simulink model "sensorless"  (R2018b)
settings: Solver=ode45  StartTime=0.0  StopTime=0.5  RelTol=1e-3  EnableMultiTasking=on
InitFcn:
  | tpwm=0.0001;
  | K=0.0604;
  | L1=0.00248;
  | L2=-1.239e-7*40;
  | Td=0;
  | kr=50;
  | wc=5;
  | speedref=10;
  | L1=0.00248;
  | L2=-1.239e-7*200;
libraries: dspsigops x72, powerlib x31, powerlib_meascontrol x24, simulink x8, powerlib_extras x5
(part 2 of 2)

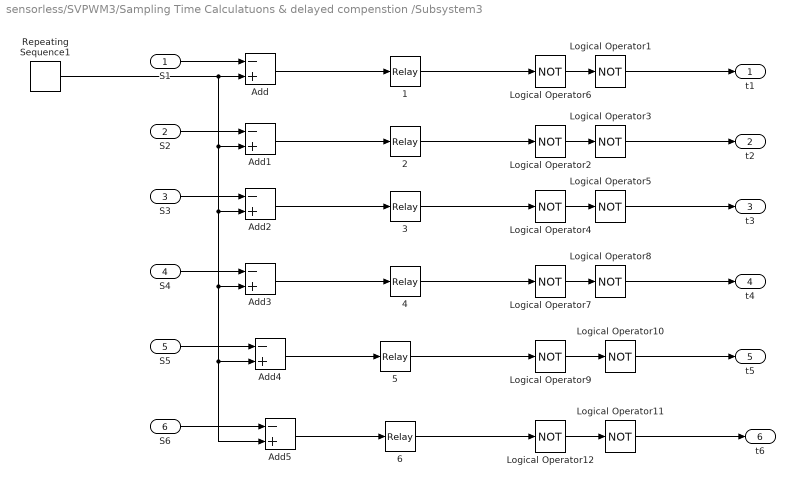
== system sensorless/SVPWM3/Sampling Time Calculatuons & delayed compenstion /Subsystem3 ==
  S1 : Inport
  S2 : Inport  Port=2
  S3 : Inport  Port=3
  S4 : Inport  Port=4
  S5 : Inport  Port=5
  S6 : Inport  Port=6
  {1..6} (6 alike) : Relay
  Add{,1..5} (6 alike) : Sum  Inputs=-+
  Logical Operator{1..12} (12 alike) : Logic  Operator=NOT  AllPortsSameDT=off  OutDataTypeStr=boolean
  Repeating Sequence1 : simulink/Sources/Repeating Sequence  rep_seq_t=[0 tpwm]  rep_seq_y=[0 tpwm]
  t1 : Outport
  t2 : Outport  Port=2
  t3 : Outport  Port=3
  t4 : Outport  Port=4
  t5 : Outport  Port=5
  t6 : Outport  Port=6
  wires:
  Add/1 -> 1/1
  1/1 -> Logical Operator6/1
  Logical Operator6/1 -> Logical Operator1/1
  Logical Operator2/1 -> Logical Operator3/1
  S1/1 -> Add/1
  S2/1 -> Add1/1
  S3/1 -> Add2/1
  Logical Operator4/1 -> Logical Operator5/1
  Add1/1 -> 2/1
  Add2/1 -> 3/1
  2/1 -> Logical Operator2/1
  3/1 -> Logical Operator4/1
  Logical Operator3/1 -> t2/1
  Logical Operator5/1 -> t3/1
  Logical Operator1/1 -> t1/1
  S4/1 -> Add3/1
  Add3/1 -> 4/1
  4/1 -> Logical Operator7/1
  Logical Operator7/1 -> Logical Operator8/1
  Logical Operator8/1 -> t4/1
  S5/1 -> Add4/1
  Add4/1 -> 5/1
  5/1 -> Logical Operator9/1
  Logical Operator9/1 -> Logical Operator10/1
  Logical Operator10/1 -> t5/1
  S6/1 -> Add5/1
  Add5/1 -> 6/1
  6/1 -> Logical Operator12/1
  Logical Operator12/1 -> Logical Operator11/1
  Logical Operator11/1 -> t6/1
  Repeating Sequence1/1 -> Add3/2, Add4/2, Add5/2, Add2/2, Add1/2, Add/2

== system sensorless/SVPWM3/Subsystem/Subsystem1 ==
  t1 : Inport
  t2 : Inport  Port=2
  tpwm : Inport  Port=3
  dt1 : Inport  Port=4
  phase currents : Inport  Port=5
  Add{,1..5} (6 alike) : Sum  Inputs=-+
  Divide{1..6} (6 alike) : Product  Inputs=*/
  PWM7 : Scope  NumInputPorts=2
  Sampled Current @ t2 : Subsystem
  Sampled Currents @ t1 : Subsystem
  Out1 : Outport
  Out2 : Outport  Port=2
  Out3 : Outport  Port=3
  Out4 : Outport  Port=4
  Out5 : Outport  Port=5
  Out6 : Outport  Port=6
  wires:
  Divide6/1 -> Out6/1
  Divide5/1 -> Out5/1
  Divide4/1 -> Out4/1
  Divide3/1 -> Out3/1
  Divide2/1 -> Out2/1
  Divide1/1 -> PWM7/1, Out1/1
  t2/1 -> Sampled Current @ t2/1(t1)
  t1/1 -> Sampled Currents @ t1/1(t1)
  phase currents/1 -> Sampled Currents @ t1/3(phase currents), Sampled Current @ t2/2(phase currents)
  tpwm/1 -> Sampled Currents @ t1/2(tpwm), Sampled Current @ t2/3(tpwm)
  dt1/1 -> Divide6/2, Divide5/2, Divide4/2, Divide3/2, Divide2/2, Divide1/2
  Add4/1 -> Divide5/1
  Add3/1 -> Divide4/1
  Sampled Current @ t2/6(Out6) -> Add5/2
  Sampled Current @ t2/2(Out2) -> Add1/2
  Add2/1 -> Divide3/1
  Sampled Currents @ t1/5(Out5) -> Add4/1
  Sampled Currents @ t1/4(Out4) -> Add3/1
  Sampled Current @ t2/5(Out5) -> Add4/2
  Add1/1 -> Divide2/1
  Sampled Current @ t2/4(Out4) -> Add3/2
  Sampled Currents @ t1/6(Out6) -> Add5/1
  Sampled Currents @ t1/1(Out1) -> Add/1
  Sampled Currents @ t1/3(Out3) -> Add2/1
  Add/1 -> Divide1/1, PWM7/2
  Sampled Current @ t2/1(Out1) -> Add/2
  Sampled Currents @ t1/2(Out2) -> Add1/1
  Add5/1 -> Divide6/1
  Sampled Current @ t2/3(Out3) -> Add2/2

== system sensorless/SVPWM3/Subsystem/Subsystem3 ==
  t1 : Inport
  t2 : Inport  Port=2
  tpwm : Inport  Port=3
  dt1 : Inport  Port=4
  phase currents : Inport  Port=5
  Add{,1..5} (6 alike) : Sum  Inputs=-+
  Divide{1..6} (6 alike) : Product  Inputs=*/
  PWM7 : Scope  NumInputPorts=2
  Sampled Current @ t2 : Subsystem
  Sampled Currents @ t1 : Subsystem
  Out1 : Outport
  Out2 : Outport  Port=2
  Out3 : Outport  Port=3
  Out4 : Outport  Port=4
  Out5 : Outport  Port=5
  Out6 : Outport  Port=6
  wires:
  Sampled Current @ t2/3(Out3) -> Add2/2
  Add5/1 -> Divide6/1
  Sampled Currents @ t1/2(Out2) -> Add1/1
  Sampled Current @ t2/1(Out1) -> Add/2
  Add/1 -> PWM7/2, Divide1/1
  Sampled Currents @ t1/3(Out3) -> Add2/1
  Sampled Currents @ t1/1(Out1) -> Add/1
  Sampled Currents @ t1/6(Out6) -> Add5/1
  Sampled Current @ t2/4(Out4) -> Add3/2
  Add1/1 -> Divide2/1
  Sampled Current @ t2/5(Out5) -> Add4/2
  Sampled Currents @ t1/4(Out4) -> Add3/1
  Sampled Currents @ t1/5(Out5) -> Add4/1
  Add2/1 -> Divide3/1
  Sampled Current @ t2/2(Out2) -> Add1/2
  Sampled Current @ t2/6(Out6) -> Add5/2
  Add3/1 -> Divide4/1
  Add4/1 -> Divide5/1
  dt1/1 -> Divide1/2, Divide2/2, Divide3/2, Divide4/2, Divide5/2, Divide6/2
  tpwm/1 -> Sampled Current @ t2/3(tpwm), Sampled Currents @ t1/2(tpwm)
  phase currents/1 -> Sampled Current @ t2/2(phase currents), Sampled Currents @ t1/3(phase currents)
  t1/1 -> Sampled Currents @ t1/1(t1)
  t2/1 -> Sampled Current @ t2/1(t1)
  Divide1/1 -> Out1/1, PWM7/1
  Divide2/1 -> Out2/1
  Divide3/1 -> Out3/1
  Divide4/1 -> Out4/1
  Divide5/1 -> Out5/1
  Divide6/1 -> Out6/1

== system sensorless/SVPWM3/Subsystem/Subsystem4 ==
  t1 : Inport
  t2 : Inport  Port=2
  tpwm : Inport  Port=3
  dt1 : Inport  Port=4
  phase currents : Inport  Port=5
  Add{,1..5} (6 alike) : Sum  Inputs=-+
  Divide{1..6} (6 alike) : Product  Inputs=*/
  PWM7 : Scope  NumInputPorts=2
  Sampled Current @ t2 : Subsystem
  Sampled Currents @ t1 : Subsystem
  Out1 : Outport
  Out2 : Outport  Port=2
  Out3 : Outport  Port=3
  Out4 : Outport  Port=4
  Out5 : Outport  Port=5
  Out6 : Outport  Port=6
  wires:
  Sampled Current @ t2/3(Out3) -> Add2/2
  Add5/1 -> Divide6/1
  Sampled Currents @ t1/2(Out2) -> Add1/1
  Sampled Current @ t2/1(Out1) -> Add/2
  Add/1 -> PWM7/2, Divide1/1
  Sampled Currents @ t1/3(Out3) -> Add2/1
  Sampled Currents @ t1/1(Out1) -> Add/1
  Sampled Currents @ t1/6(Out6) -> Add5/1
  Sampled Current @ t2/4(Out4) -> Add3/2
  Add1/1 -> Divide2/1
  Sampled Current @ t2/5(Out5) -> Add4/2
  Sampled Currents @ t1/4(Out4) -> Add3/1
  Sampled Currents @ t1/5(Out5) -> Add4/1
  Add2/1 -> Divide3/1
  Sampled Current @ t2/2(Out2) -> Add1/2
  Sampled Current @ t2/6(Out6) -> Add5/2
  Add3/1 -> Divide4/1
  Add4/1 -> Divide5/1
  dt1/1 -> Divide1/2, Divide2/2, Divide3/2, Divide4/2, Divide5/2, Divide6/2
  tpwm/1 -> Sampled Current @ t2/3(tpwm), Sampled Currents @ t1/2(tpwm)
  phase currents/1 -> Sampled Current @ t2/2(phase currents), Sampled Currents @ t1/3(phase currents)
  t1/1 -> Sampled Currents @ t1/1(t1)
  t2/1 -> Sampled Current @ t2/1(t1)
  Divide1/1 -> Out1/1, PWM7/1
  Divide2/1 -> Out2/1
  Divide3/1 -> Out3/1
  Divide4/1 -> Out4/1
  Divide5/1 -> Out5/1
  Divide6/1 -> Out6/1

== system sensorless/dq-sixphasePMSM/dynamics/Theta Generator (-pi, pi) ==
  pi : Inport
  In : Inport  Port=2
  Compare To Constant : simulink/Logic and Bit Operations/Compare To Constant  relop=>  const=pi/2  OutDataTypeStr=uint8  ZeroCross=off
  Constant3 : Constant  Value=0
  Sum2 : Sum  Inputs=+-
  Switch : Switch  Threshold=0.5
  Out : Outport
  wires:
  Compare To Constant/1 -> Switch/2
  Switch/1 -> Sum2/2
  Constant3/1 -> Switch/3
  pi/1 -> Switch/1
  In/1 -> Sum2/1, Compare To Constant/1
  Sum2/1 -> Out/1

== system sensorless/dq-sixphasePMSM/z-p/Subsystem ==
  Phase : Inport
  La0 : Constant  Value=-0.00139e-3
  La1 : Constant  Value=1.5201e-3
  La2 : Constant  Value=0.54985e-3
  Ldq_dmm1 : Scope  NumInputPorts=6
  Lg0 : Constant  Value=-0.0000798e-3
  Lg1 : Constant  Value=-0.000032e-3
  Lg2 : Constant  Value=-0.000052e-3
  "Manually Calculated Results " : MATLAB Function  TreatAsAtomicUnit=on
  Lz1 : Outport
  Lz2 : Outport  Port=2
  Lz1z2 : Outport  Port=3
  wires:
  "Manually Calculated Results "/3(Lz1) -> Lz1/1, Ldq_dmm1/3
  Lg2/1 -> "Manually Calculated Results "/6(Lg2)
  Lg1/1 -> "Manually Calculated Results "/5(Lg1)
  "Manually Calculated Results "/2(Lq) -> Ldq_dmm1/2
  Lg0/1 -> "Manually Calculated Results "/3(Lg0)
  "Manually Calculated Results "/4(Lz2) -> Lz2/1, Ldq_dmm1/4
  "Manually Calculated Results "/1(Ld) -> Ldq_dmm1/1
  "Manually Calculated Results "/5(Lz1z2) -> Lz1z2/1, Ldq_dmm1/5
  La0/1 -> "Manually Calculated Results "/1(La0)
  La1/1 -> "Manually Calculated Results "/2(La1)
  La2/1 -> "Manually Calculated Results "/4(La2)
  Phase/1 -> "Manually Calculated Results "/7(RP)

== system sensorless/dq-sixphasePMSM/z-p1/Subsystem ==
  Phase : Inport
  La0 : Constant  Value=-0.00139e-3
  La1 : Constant  Value=1.5201e-3
  La2 : Constant  Value=0.54985e-3
  Ldq_dmm1 : Scope  NumInputPorts=3
  Lg0 : Constant  Value=-0.0000798e-3
  Lg1 : Constant  Value=-0.000032e-3
  Lg2 : Constant  Value=-0.000052e-3
  "Manually Calculated Results " : MATLAB Function  TreatAsAtomicUnit=on
  Lalpha : Outport
  Lbeta : Outport  Port=2
  Lalpha_beta : Outport  Port=3
  wires:
  Lg2/1 -> "Manually Calculated Results "/6(Lg2)
  Lg1/1 -> "Manually Calculated Results "/5(Lg1)
  "Manually Calculated Results "/2(Lbeta) -> Ldq_dmm1/2, Lbeta/1
  Lg0/1 -> "Manually Calculated Results "/3(Lg0)
  "Manually Calculated Results "/1(Lalpha) -> Lalpha/1, Ldq_dmm1/1
  La0/1 -> "Manually Calculated Results "/1(La0)
  La1/1 -> "Manually Calculated Results "/2(La1)
  La2/1 -> "Manually Calculated Results "/4(La2)
  Phase/1 -> "Manually Calculated Results "/7(RP)
  "Manually Calculated Results "/3(Lalphabeta) -> Ldq_dmm1/3, Lalpha_beta/1

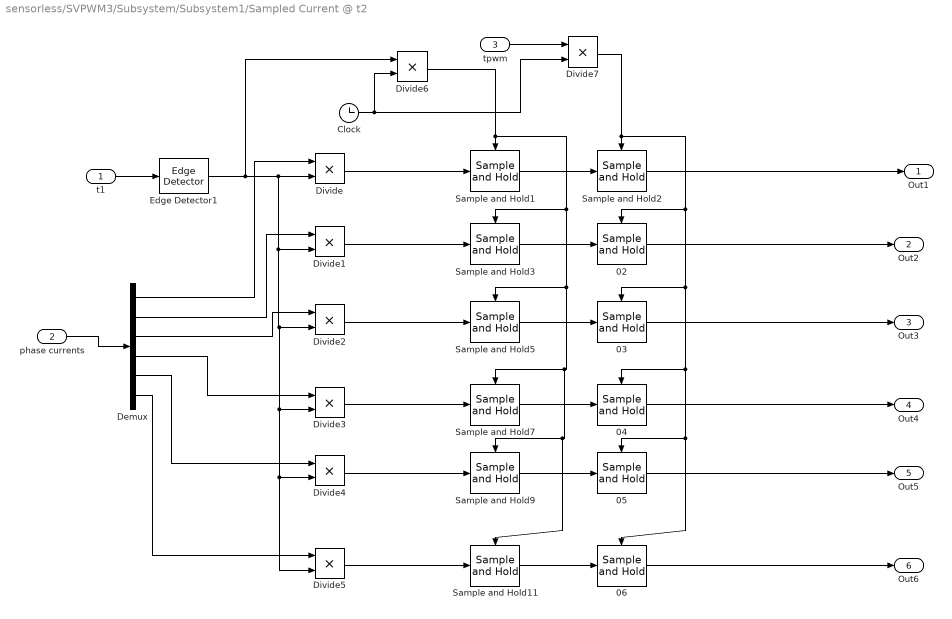
== system sensorless/SVPWM3/Subsystem/Subsystem1/Sampled Current @ t2 ==
  t1 : Inport
  phase currents : Inport  Port=2
  tpwm : Inport  Port=3
  02 : dspsigops/Sample and Hold  trig=Rising edge  initCond=0  latchinput=off
  03 : dspsigops/Sample and Hold  trig=Rising edge  initCond=0  latchinput=off
  04 : dspsigops/Sample and Hold  trig=Rising edge  initCond=0  latchinput=off
  "05 " : dspsigops/Sample and Hold  trig=Rising edge  initCond=0  latchinput=off
  06 : dspsigops/Sample and Hold  trig=Rising edge  initCond=0  latchinput=off
  Clock : Clock
  Demux : Demux  Outputs=6
  Divide{,1..7} (8 alike) : Product  Inputs=**
  Edge Detector1 : powerlib_meascontrol/Logic/Edge Detector  model=Rising  ic=0  Ts=0
      settings: SourceProductName=Simscape Power Systems  SourceProductBaseCode=PS
  Sample and Hold{1..3,5,7,9,11} (7 alike) : dspsigops/Sample and Hold  trig=Rising edge  initCond=0  latchinput=off
  Out1 : Outport
  Out2 : Outport  Port=2
  Out3 : Outport  Port=3
  Out4 : Outport  Port=4
  Out5 : Outport  Port=5
  Out6 : Outport  Port=6
  wires:
  Divide6/1 -> Sample and Hold11/Trigger, Sample and Hold9/Trigger, Sample and Hold7/Trigger, Sample and Hold5/Trigger, Sample and Hold3/Trigger, Sample and Hold1/Trigger
  06/1 -> Out6/1
  "05 "/1 -> Out5/1
  04/1 -> Out4/1
  03/1 -> Out3/1
  02/1 -> Out2/1
  Sample and Hold2/1 -> Out1/1
  Sample and Hold1/1 -> Sample and Hold2/1
  Edge Detector1/1 -> Divide6/1, Divide5/2, Divide4/2, Divide3/2, Divide2/2, Divide1/2, Divide/2
  Divide/1 -> Sample and Hold1/1
  t1/1 -> Edge Detector1/1
  Clock/1 -> Divide7/2, Divide6/2
  Divide7/1 -> 02/Trigger, 03/Trigger, 04/Trigger, "05 "/Trigger, 06/Trigger, Sample and Hold2/Trigger
  tpwm/1 -> Divide7/1
  Divide1/1 -> Sample and Hold3/1
  Sample and Hold3/1 -> 02/1
  Divide2/1 -> Sample and Hold5/1
  Sample and Hold5/1 -> 03/1
  Divide3/1 -> Sample and Hold7/1
  Sample and Hold7/1 -> 04/1
  Divide4/1 -> Sample and Hold9/1
  Sample and Hold9/1 -> "05 "/1
  Divide5/1 -> Sample and Hold11/1
  Sample and Hold11/1 -> 06/1
  phase currents/1 -> Demux/1
  Demux/1 -> Divide/1
  Demux/2 -> Divide1/1
  Demux/3 -> Divide2/1
  Demux/4 -> Divide3/1
  Demux/5 -> Divide4/1
  Demux/6 -> Divide5/1

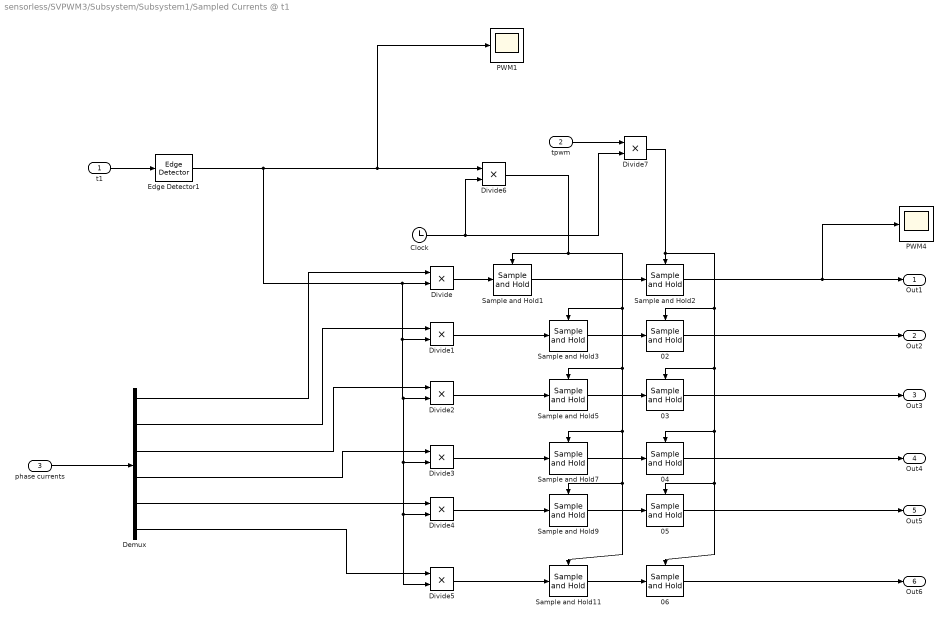
== system sensorless/SVPWM3/Subsystem/Subsystem1/Sampled Currents @ t1 ==
  t1 : Inport
  tpwm : Inport  Port=2
  phase currents : Inport  Port=3
  02 : dspsigops/Sample and Hold  trig=Rising edge  initCond=0  latchinput=off
  03 : dspsigops/Sample and Hold  trig=Rising edge  initCond=0  latchinput=off
  04 : dspsigops/Sample and Hold  trig=Rising edge  initCond=0  latchinput=off
  "05 " : dspsigops/Sample and Hold  trig=Rising edge  initCond=0  latchinput=off
  06 : dspsigops/Sample and Hold  trig=Rising edge  initCond=0  latchinput=off
  Clock : Clock
  Demux : Demux  Outputs=6
  Divide{,1..7} (8 alike) : Product  Inputs=**
  Edge Detector1 : powerlib_meascontrol/Logic/Edge Detector  model=Rising  ic=0  Ts=0
      settings: SourceProductName=Simscape Power Systems  SourceProductBaseCode=PS
  PWM1 : Scope
  PWM4 : Scope
  Sample and Hold{1..3,5,7,9,11} (7 alike) : dspsigops/Sample and Hold  trig=Rising edge  initCond=0  latchinput=off
  Out1 : Outport
  Out2 : Outport  Port=2
  Out3 : Outport  Port=3
  Out4 : Outport  Port=4
  Out5 : Outport  Port=5
  Out6 : Outport  Port=6
  wires:
  06/1 -> Out6/1
  "05 "/1 -> Out5/1
  04/1 -> Out4/1
  03/1 -> Out3/1
  02/1 -> Out2/1
  Sample and Hold2/1 -> PWM4/1, Out1/1
  Sample and Hold1/1 -> Sample and Hold2/1
  Divide/1 -> Sample and Hold1/1
  t1/1 -> Edge Detector1/1
  Clock/1 -> Divide6/2, Divide7/2
  Divide6/1 -> Sample and Hold11/Trigger, Sample and Hold9/Trigger, Sample and Hold7/Trigger, Sample and Hold5/Trigger, Sample and Hold3/Trigger, Sample and Hold1/Trigger
  tpwm/1 -> Divide7/1
  Divide1/1 -> Sample and Hold3/1
  Sample and Hold3/1 -> 02/1
  Divide2/1 -> Sample and Hold5/1
  Sample and Hold5/1 -> 03/1
  Divide3/1 -> Sample and Hold7/1
  Sample and Hold7/1 -> 04/1
  Divide4/1 -> Sample and Hold9/1
  Sample and Hold9/1 -> "05 "/1
  Divide5/1 -> Sample and Hold11/1
  Sample and Hold11/1 -> 06/1
  phase currents/1 -> Demux/1
  Demux/1 -> Divide/1
  Demux/2 -> Divide1/1
  Demux/3 -> Divide2/1
  Demux/4 -> Divide3/1
  Demux/5 -> Divide4/1
  Demux/6 -> Divide5/1
  Divide7/1 -> 02/Trigger, 03/Trigger, 04/Trigger, "05 "/Trigger, 06/Trigger, Sample and Hold2/Trigger
  Edge Detector1/1 -> Divide5/2, Divide4/2, Divide3/2, Divide2/2, Divide1/2, Divide/2, Divide6/1, PWM1/1

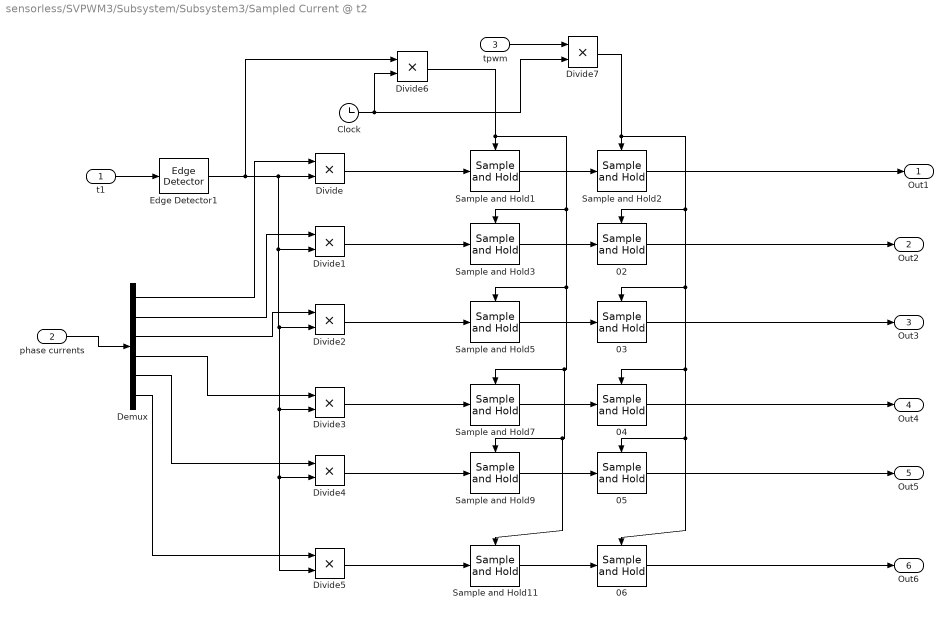
== system sensorless/SVPWM3/Subsystem/Subsystem3/Sampled Current @ t2 ==
  t1 : Inport
  phase currents : Inport  Port=2
  tpwm : Inport  Port=3
  02 : dspsigops/Sample and Hold  trig=Rising edge  initCond=0  latchinput=off
  03 : dspsigops/Sample and Hold  trig=Rising edge  initCond=0  latchinput=off
  04 : dspsigops/Sample and Hold  trig=Rising edge  initCond=0  latchinput=off
  "05 " : dspsigops/Sample and Hold  trig=Rising edge  initCond=0  latchinput=off
  06 : dspsigops/Sample and Hold  trig=Rising edge  initCond=0  latchinput=off
  Clock : Clock
  Demux : Demux  Outputs=6
  Divide{,1..7} (8 alike) : Product  Inputs=**
  Edge Detector1 : powerlib_meascontrol/Logic/Edge Detector  model=Rising  ic=0  Ts=0
      settings: SourceProductName=Simscape Power Systems  SourceProductBaseCode=PS
  Sample and Hold{1..3,5,7,9,11} (7 alike) : dspsigops/Sample and Hold  trig=Rising edge  initCond=0  latchinput=off
  Out1 : Outport
  Out2 : Outport  Port=2
  Out3 : Outport  Port=3
  Out4 : Outport  Port=4
  Out5 : Outport  Port=5
  Out6 : Outport  Port=6
  wires:
  Demux/6 -> Divide5/1
  Demux/5 -> Divide4/1
  Demux/4 -> Divide3/1
  Demux/3 -> Divide2/1
  Demux/2 -> Divide1/1
  Demux/1 -> Divide/1
  phase currents/1 -> Demux/1
  Sample and Hold11/1 -> 06/1
  Divide5/1 -> Sample and Hold11/1
  Sample and Hold9/1 -> "05 "/1
  Divide4/1 -> Sample and Hold9/1
  Sample and Hold7/1 -> 04/1
  Divide3/1 -> Sample and Hold7/1
  Sample and Hold5/1 -> 03/1
  Divide2/1 -> Sample and Hold5/1
  Sample and Hold3/1 -> 02/1
  Divide1/1 -> Sample and Hold3/1
  tpwm/1 -> Divide7/1
  Divide7/1 -> Sample and Hold2/Trigger, 06/Trigger, "05 "/Trigger, 04/Trigger, 03/Trigger, 02/Trigger
  Clock/1 -> Divide6/2, Divide7/2
  t1/1 -> Edge Detector1/1
  Divide/1 -> Sample and Hold1/1
  Edge Detector1/1 -> Divide/2, Divide1/2, Divide2/2, Divide3/2, Divide4/2, Divide5/2, Divide6/1
  Sample and Hold1/1 -> Sample and Hold2/1
  Sample and Hold2/1 -> Out1/1
  02/1 -> Out2/1
  03/1 -> Out3/1
  04/1 -> Out4/1
  "05 "/1 -> Out5/1
  06/1 -> Out6/1
  Divide6/1 -> Sample and Hold1/Trigger, Sample and Hold3/Trigger, Sample and Hold5/Trigger, Sample and Hold7/Trigger, Sample and Hold9/Trigger, Sample and Hold11/Trigger

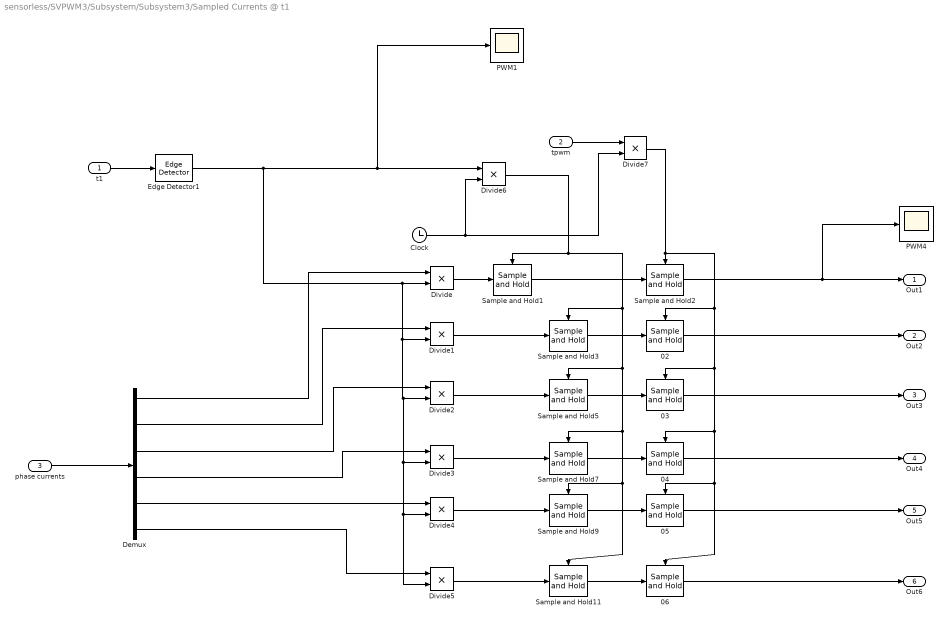
== system sensorless/SVPWM3/Subsystem/Subsystem3/Sampled Currents @ t1 ==
  t1 : Inport
  tpwm : Inport  Port=2
  phase currents : Inport  Port=3
  02 : dspsigops/Sample and Hold  trig=Rising edge  initCond=0  latchinput=off
  03 : dspsigops/Sample and Hold  trig=Rising edge  initCond=0  latchinput=off
  04 : dspsigops/Sample and Hold  trig=Rising edge  initCond=0  latchinput=off
  "05 " : dspsigops/Sample and Hold  trig=Rising edge  initCond=0  latchinput=off
  06 : dspsigops/Sample and Hold  trig=Rising edge  initCond=0  latchinput=off
  Clock : Clock
  Demux : Demux  Outputs=6
  Divide{,1..7} (8 alike) : Product  Inputs=**
  Edge Detector1 : powerlib_meascontrol/Logic/Edge Detector  model=Rising  ic=0  Ts=0
      settings: SourceProductName=Simscape Power Systems  SourceProductBaseCode=PS
  PWM1 : Scope
  PWM4 : Scope
  Sample and Hold{1..3,5,7,9,11} (7 alike) : dspsigops/Sample and Hold  trig=Rising edge  initCond=0  latchinput=off
  Out1 : Outport
  Out2 : Outport  Port=2
  Out3 : Outport  Port=3
  Out4 : Outport  Port=4
  Out5 : Outport  Port=5
  Out6 : Outport  Port=6
  wires:
  Edge Detector1/1 -> PWM1/1, Divide6/1, Divide/2, Divide1/2, Divide2/2, Divide3/2, Divide4/2, Divide5/2
  Divide7/1 -> Sample and Hold2/Trigger, 06/Trigger, "05 "/Trigger, 04/Trigger, 03/Trigger, 02/Trigger
  Demux/6 -> Divide5/1
  Demux/5 -> Divide4/1
  Demux/4 -> Divide3/1
  Demux/3 -> Divide2/1
  Demux/2 -> Divide1/1
  Demux/1 -> Divide/1
  phase currents/1 -> Demux/1
  Sample and Hold11/1 -> 06/1
  Divide5/1 -> Sample and Hold11/1
  Sample and Hold9/1 -> "05 "/1
  Divide4/1 -> Sample and Hold9/1
  Sample and Hold7/1 -> 04/1
  Divide3/1 -> Sample and Hold7/1
  Sample and Hold5/1 -> 03/1
  Divide2/1 -> Sample and Hold5/1
  Sample and Hold3/1 -> 02/1
  Divide1/1 -> Sample and Hold3/1
  tpwm/1 -> Divide7/1
  Divide6/1 -> Sample and Hold1/Trigger, Sample and Hold3/Trigger, Sample and Hold5/Trigger, Sample and Hold7/Trigger, Sample and Hold9/Trigger, Sample and Hold11/Trigger
  Clock/1 -> Divide7/2, Divide6/2
  t1/1 -> Edge Detector1/1
  Divide/1 -> Sample and Hold1/1
  Sample and Hold1/1 -> Sample and Hold2/1
  Sample and Hold2/1 -> Out1/1, PWM4/1
  02/1 -> Out2/1
  03/1 -> Out3/1
  04/1 -> Out4/1
  "05 "/1 -> Out5/1
  06/1 -> Out6/1

== system sensorless/SVPWM3/Subsystem/Subsystem4/Sampled Current @ t2 ==
  t1 : Inport
  phase currents : Inport  Port=2
  tpwm : Inport  Port=3
  02 : dspsigops/Sample and Hold  trig=Rising edge  initCond=0  latchinput=off
  03 : dspsigops/Sample and Hold  trig=Rising edge  initCond=0  latchinput=off
  04 : dspsigops/Sample and Hold  trig=Rising edge  initCond=0  latchinput=off
  "05 " : dspsigops/Sample and Hold  trig=Rising edge  initCond=0  latchinput=off
  06 : dspsigops/Sample and Hold  trig=Rising edge  initCond=0  latchinput=off
  Clock : Clock
  Demux : Demux  Outputs=6
  Divide{,1..7} (8 alike) : Product  Inputs=**
  Edge Detector1 : powerlib_meascontrol/Logic/Edge Detector  model=Rising  ic=0  Ts=0
      settings: SourceProductName=Simscape Power Systems  SourceProductBaseCode=PS
  Sample and Hold{1..3,5,7,9,11} (7 alike) : dspsigops/Sample and Hold  trig=Rising edge  initCond=0  latchinput=off
  Out1 : Outport
  Out2 : Outport  Port=2
  Out3 : Outport  Port=3
  Out4 : Outport  Port=4
  Out5 : Outport  Port=5
  Out6 : Outport  Port=6
  wires:
  Demux/6 -> Divide5/1
  Demux/5 -> Divide4/1
  Demux/4 -> Divide3/1
  Demux/3 -> Divide2/1
  Demux/2 -> Divide1/1
  Demux/1 -> Divide/1
  phase currents/1 -> Demux/1
  Sample and Hold11/1 -> 06/1
  Divide5/1 -> Sample and Hold11/1
  Sample and Hold9/1 -> "05 "/1
  Divide4/1 -> Sample and Hold9/1
  Sample and Hold7/1 -> 04/1
  Divide3/1 -> Sample and Hold7/1
  Sample and Hold5/1 -> 03/1
  Divide2/1 -> Sample and Hold5/1
  Sample and Hold3/1 -> 02/1
  Divide1/1 -> Sample and Hold3/1
  tpwm/1 -> Divide7/1
  Divide7/1 -> Sample and Hold2/Trigger, 06/Trigger, "05 "/Trigger, 04/Trigger, 03/Trigger, 02/Trigger
  Clock/1 -> Divide6/2, Divide7/2
  t1/1 -> Edge Detector1/1
  Divide/1 -> Sample and Hold1/1
  Edge Detector1/1 -> Divide/2, Divide1/2, Divide2/2, Divide3/2, Divide4/2, Divide5/2, Divide6/1
  Sample and Hold1/1 -> Sample and Hold2/1
  Sample and Hold2/1 -> Out1/1
  02/1 -> Out2/1
  03/1 -> Out3/1
  04/1 -> Out4/1
  "05 "/1 -> Out5/1
  06/1 -> Out6/1
  Divide6/1 -> Sample and Hold1/Trigger, Sample and Hold3/Trigger, Sample and Hold5/Trigger, Sample and Hold7/Trigger, Sample and Hold9/Trigger, Sample and Hold11/Trigger

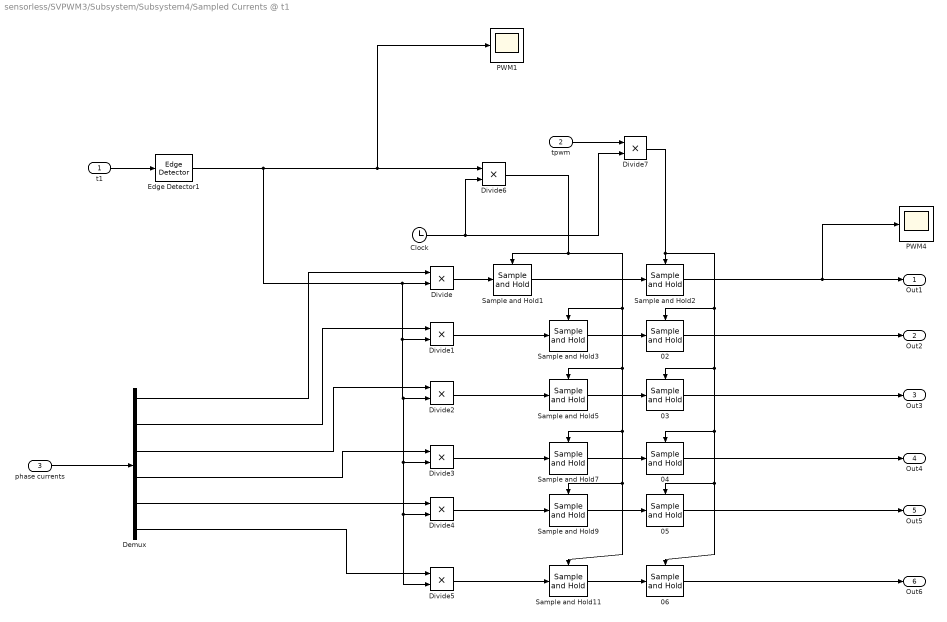
== system sensorless/SVPWM3/Subsystem/Subsystem4/Sampled Currents @ t1 ==
  t1 : Inport
  tpwm : Inport  Port=2
  phase currents : Inport  Port=3
  02 : dspsigops/Sample and Hold  trig=Rising edge  initCond=0  latchinput=off
  03 : dspsigops/Sample and Hold  trig=Rising edge  initCond=0  latchinput=off
  04 : dspsigops/Sample and Hold  trig=Rising edge  initCond=0  latchinput=off
  "05 " : dspsigops/Sample and Hold  trig=Rising edge  initCond=0  latchinput=off
  06 : dspsigops/Sample and Hold  trig=Rising edge  initCond=0  latchinput=off
  Clock : Clock
  Demux : Demux  Outputs=6
  Divide{,1..7} (8 alike) : Product  Inputs=**
  Edge Detector1 : powerlib_meascontrol/Logic/Edge Detector  model=Rising  ic=0  Ts=0
      settings: SourceProductName=Simscape Power Systems  SourceProductBaseCode=PS
  PWM1 : Scope
  PWM4 : Scope
  Sample and Hold{1..3,5,7,9,11} (7 alike) : dspsigops/Sample and Hold  trig=Rising edge  initCond=0  latchinput=off
  Out1 : Outport
  Out2 : Outport  Port=2
  Out3 : Outport  Port=3
  Out4 : Outport  Port=4
  Out5 : Outport  Port=5
  Out6 : Outport  Port=6
  wires:
  Edge Detector1/1 -> PWM1/1, Divide6/1, Divide/2, Divide1/2, Divide2/2, Divide3/2, Divide4/2, Divide5/2
  Divide7/1 -> Sample and Hold2/Trigger, 06/Trigger, "05 "/Trigger, 04/Trigger, 03/Trigger, 02/Trigger
  Demux/6 -> Divide5/1
  Demux/5 -> Divide4/1
  Demux/4 -> Divide3/1
  Demux/3 -> Divide2/1
  Demux/2 -> Divide1/1
  Demux/1 -> Divide/1
  phase currents/1 -> Demux/1
  Sample and Hold11/1 -> 06/1
  Divide5/1 -> Sample and Hold11/1
  Sample and Hold9/1 -> "05 "/1
  Divide4/1 -> Sample and Hold9/1
  Sample and Hold7/1 -> 04/1
  Divide3/1 -> Sample and Hold7/1
  Sample and Hold5/1 -> 03/1
  Divide2/1 -> Sample and Hold5/1
  Sample and Hold3/1 -> 02/1
  Divide1/1 -> Sample and Hold3/1
  tpwm/1 -> Divide7/1
  Divide6/1 -> Sample and Hold1/Trigger, Sample and Hold3/Trigger, Sample and Hold5/Trigger, Sample and Hold7/Trigger, Sample and Hold9/Trigger, Sample and Hold11/Trigger
  Clock/1 -> Divide7/2, Divide6/2
  t1/1 -> Edge Detector1/1
  Divide/1 -> Sample and Hold1/1
  Sample and Hold1/1 -> Sample and Hold2/1
  Sample and Hold2/1 -> Out1/1, PWM4/1
  02/1 -> Out2/1
  03/1 -> Out3/1
  04/1 -> Out4/1
  "05 "/1 -> Out5/1
  06/1 -> Out6/1

== matlab function sensorless/clark1 ==
  data: Ualpha output; Ua input; Ubeta output; Ub input; Uc input; Uu input; Uv input; Uz1 output; Uz2 output; Uz3 output; Uz4 output; Uw input
function [Ualpha,Ubeta,Uz1,Uz2,Uz3,Uz4] = clark(Ua,Ub,Uc,Uu,Uv,Uw)

T=1/sqrt(3)*[1,  (-1/2),    (-1/2),       sqrt(3)/2,  -sqrt(3)/2,  0;
       0,  sqrt(3)/2, (-sqrt(3)/2), 1/2,        1/2,        -1;
       1,  (-1/2),    (-1/2),       -sqrt(3)/2, sqrt(3)/2,   0;
       0,  -sqrt(3)/2,sqrt(3)/2,    1/2,        1/2,        -1;
       1,  1,         1,            0,          0,           0;
       0,  0,         0,            1,          1,           1];
X=[Ua;Ub;Uc;Uu;Uv;Uw];
Y=T*X;
Ualpha=Y(1);
Ubeta=Y(2);
Uz1=Y(3);
Uz2=Y(4);
Uz3=Y(5);
Uz4=Y(6);
end

== matlab function sensorless/Embedded MATLAB Function ==
  data: uo output; uab input; ua output; ubc input; ucd input; ude input; uef input; ub output; uc output; ud output; ue output; uf output
function [uo,ua,ub,uc,ud,ue,uf] = fcn(uab,ubc,ucd,ude,uef)

%#eml
uxx=[uab,ubc,ucd,ude,uef,0,0]';
T=1/6*[2 0 2 0 2 -2 2;
4 4 2 2 0 2 0;
0 4 4 2 2 0 2;
-2 -2 2 2 0 2 0;
0 -2 -2 2 2 0 2;
-2 -2 -4 -4 0 2 0;
0 -2 -2 -4 -4 0 2];
I=T*uxx;
uo=I(1);
ua=I(2);
ub=I(3);
uc=I(4);
ud=I(5);
ue=I(6);
uf=I(7);

== matlab function sensorless/SVPWM3/Sampling Time Calculatuons & delayed compenstion /Embedded MATLAB Function1 ==
  data: N input; T1 input; T2 input; T3 input; T4 input; T0 input; t1 output; t2 output; t3 output; t4 output; t5 output; t6 output
function [t1,t2,t3,t4,t5,t6] = fcn(N,T1,T2,T3,T4,T0)

%#xsxx
Ta=T0/4;
Tb=Ta+T2;
Tc=Tb+T1;
Td=Tc+T0/2;
Te=Td+T4;
Tf=Te+T3;
Ta1=T0/4;
Tb1=Ta1+T1;
Tc1=Tb1+T2;
Td1=Tc1+T0/2;
Te1=Td1+T3;
Tf1=Te1+T4;
    t1=0;
    t2=0;
    t3=0;
    t4=0;
    t5=0;
    t6=0;
    d=1e-6;
if N==1
    t1=Ta+d;%Tcma1
    t2=Ta+14*d;%Tcme1
    t3=Tb+d;
    t4=Tb+14*d;
    t5=Tc+d;
    t6=Tc+14*d;
end
if N==2
    t1=Ta+d;%Tcma1
    t2=Ta+14*d;%Tcme1
    t3=Tb+d;
    t4=Tb+14*d;
    t5=Tc+d;
    t6=Tc+14*d;
end
if N==3
    t1=Ta1+d;%Tcma1
    t2=Ta1+14*d;%Tcme1
    t3=Tb1+d;
    t4=Tb1+14*d;
    t5=Tc1+d;
    t6=Tc1+14*d;
end
if N==4
   t1=Ta1+d;%Tcma1
    t2=Ta1+14*d;%Tcme1
    t3=Tb1+d;
    t4=Tb1+14*d;
    t5=Tc1+d;
    t6=Tc1+14*d;
end
if N==5
    t1=Ta+d;%Tcma1
    t2=Ta+14*d;%Tcme1
    t3=Tb+d;
    t4=Tb+14*d;
    t5=Tc+d;
    t6=Tc+14*d;
end
if N==6
    t1=Ta+d;%Tcma1
    t2=Ta+14*d;%Tcme1
    t3=Tb+d;
    t4=Tb+14*d;
    t5=Tc+d;
    t6=Tc+14*d;
end
if N==7
   t1=Ta1+d;%Tcma1
    t2=Ta1+14*d;%Tcme1
    t3=Tb1+d;
    t4=Tb1+14*d;
    t5=Tc1+d;
    t6=Tc1+14*d;
end
if N==8
   t1=Ta1+d;%Tcma1
    t2=Ta1+14*d;%Tcme1
    t3=Tb1+d;
    t4=Tb1+14*d;
    t5=Tc1+d;
    t6=Tc1+14*d;
end
if N==9
    t1=Ta+d;%Tcma1
    t2=Ta+14*d;%Tcme1
    t3=Tb+d;
    t4=Tb+14*d;
    t5=Tc+d;
    t6=Tc+14*d;
end
if N==10
    t1=Ta+d;%Tcma1
    t2=Ta+14*d;%Tcme1
    t3=Tb+d;
    t4=Tb+14*d;
    t5=Tc+d;
    t6=Tc+14*d;
end
if N==11
    t1=Ta1+d;%Tcma1
    t2=Ta1+14*d;%Tcme1
    t3=Tb1+d;
    t4=Tb1+14*d;
    t5=Tc1+d;
    t6=Tc1+14*d;
end
if N==12
    t1=Ta1+d;%Tcma1
    t2=Ta1+14*d;%Tcme1
    t3=Tb1+d;
    t4=Tb1+14*d;
    t5=Tc1+d;
    t6=Tc1+14*d;
end

== matlab function sensorless/SVPWM3/Sampling Time Calculatuons & delayed compenstion /Embedded MATLAB Function2 ==
  data: t1 input; t2 input; t3 input; t4 input; t5 input; t6 input; dt1 output; dt2 output; dt3 output
function [dt1,dt2,dt3] = fcn(t1,t2,t3,t4,t5,t6)

dt1=t2-t1;
dt2=t4-t3;
dt3=t6-t5;
end

== matlab function sensorless/SVPWM3/Subsystem/frame Transformation for V1 abc-alpha_beta1 ==
  data: ia input; I_alpha_dV1 output; I_beta_dV1 output; ib input; ic input; id input; ie input; if1 input
function [I_alpha_dV1,I_beta_dV1]= fcn(ia,ib,ic,id,ie,if1)
%#codegen
d=[ia,ib,ic,id,ie,if1]';
C=1/sqrt(3)*[1 sqrt(3)/2 -1/2 -sqrt(3)/2 -1/2 0;
    0 1/2 sqrt(3)/2 1/2 -sqrt(3)/2 -1;
    1 -sqrt(3)/2 -1/2 sqrt(3)/2 -1/2 0;
    0 1/2 -sqrt(3)/2 1/2 sqrt(3)/2 -1;
    1 0 1 0 1 0;
    0 1 0 1 0 1];
h=C*d;
I_alpha_dV1=h(1,1);
I_beta_dV1=h(2,1);

== matlab function sensorless/dq-sixphasePMSM/Embedded MATLAB Function1 ==
  data: ualpha output; ua input; ub input; uc input; ud input; ue input; uf input; ubeta output
function [ualpha,ubeta] = fcn(ua,ub,uc,ud,ue,uf)

%#eml
uxx=[ua,ub,uc,ud,ue,uf]';
T=1/sqrt(3)*[1 sqrt(3)/2 -1/2 -sqrt(3)/2 -1/2 0;
    0 1/2 sqrt(3)/2 1/2 -sqrt(3)/2 -1;
    1 -sqrt(3)/2 -1/2 sqrt(3)/2 -1/2 0;
    0 1/2 -sqrt(3)/2 1/2 sqrt(3)/2 -1;
    1 0 1 0 1 0;
    0 1 0 1 0 1];
I=T*uxx;
ualpha=I(1);
ubeta=I(2);

== matlab function sensorless/SVPWM3/Calculated Voltages /V_alpha2 & V_beta2 ==
  data: udc input; u_alpha2 output; u_beta2 output; N input
function [u_alpha2,u_beta2]= fcn(udc,N)
% #codegen
va01=0;
va02=0;
va03=0;
va04=0;
va05=0;
va06=0;
va07=0;
va08=0;
va09=0;
va10=0;
va11=0;
va12=0;
vb01=0;%V51
vb02=0;%V49
vb03=0;%V48
vb04=0;%60
vb05=0;%V60
vb06=0;%V28
vb07=0;%V14
vb08=0;%V15
vb09=0;%V15
vb10=0;%V07
vb11=0;%V35
vb12=0;%V51
u_alpha2=0;
u_beta2=0;
if N==1
va01=udc*1.115355072*cosd(315); 
vb01=udc*1.115355072*sind(315);
u_alpha2=va01;
u_beta2=vb01;
end
if N==2
va02=udc*1.115355072*cosd(345);
vb02=udc*1.115355072*sind(345);
u_alpha2=va02;
u_beta2=vb02;
end 
if N==3
va03=udc*1.115355072*cosd(45);
vb03=udc*1.115355072*sind(45);
u_alpha2=va03;
u_beta2=vb03;
end
if N==4
va04=udc*1.115355072*cosd(75);
vb04=udc*1.115355072*sind(75);
u_alpha2=va04;
u_beta2=vb04;
end
if N==5
va05=udc*1.115355072*cosd(75);
vb05=udc*1.115355072*sind(75);
u_alpha2=va05;
u_beta2=vb05;
end
if N==6
va06=udc*1.115355072*cosd(105);
vb06=udc*1.115355072*sind(105);
u_alpha2=va06;
u_beta2=vb06;
end
if N==7
va07=udc*1.115355072*cosd(165);
vb07=udc*1.115355072*sind(165);
u_alpha2=va07;
u_beta2=vb07;
end
if N==8
va08=udc*1.115355072*cosd(195);
vb08=udc*1.115355072*sind(195);
u_alpha2=va08;
u_beta2=vb08;
end
if N==9
va09=udc*1.115355072*cosd(195);
vb09=udc*1.115355072*sind(195);
u_alpha2=va09;
u_beta2=vb09;
end
if N==10
va10=udc*1.115355072*cosd(225);
vb10=udc*1.115355072*sind(225);
u_alpha2=va10;
u_beta2=vb10;
end
if N==11
va11=udc*1.115355072*cosd(285);
vb11=udc*1.115355072*sind(285);
u_alpha2=va11;
u_beta2=vb11;
end 
if N==12
va12=udc*1.115355072*cosd(315);
vb12=udc*1.115355072*sind(315);
u_alpha2=va12;
u_beta2=vb12;
end

== matlab function sensorless/SVPWM3/MATLAB Function3 ==
  data: x input; y output; clock input
function y = fcn(x,clock)
%#codegen

if clock<0.006
    y=0;
else
    y=x;
end
end

== matlab function sensorless/SVPWM3/SLVC_Algorithm ==
  data: i1 input; i2 input; i3 input; i4 input; i01 input; i02 input; v1 input; v2 input; v3 input; v4 input; cos output; sin output; L1 input; L2 input

function [cos,sin]  = SLVC(i1,i2,i3,i4,i01,i02,v1,v2,v3,v4,L1,L2)
%#xsxx
% %# With Out Inclusion of Zero Vector %%
% A=[(v3^2/v4)-v4,(i3)-((v3/v4)*(i4));(v1^2/v2)-v2,(i1)-((v1/v2)*(i2))];
% B=[2*v3,(i3)-((v3/v4)*(i4));2*v1,(i1)-((v1/v2)*(i2))];
% C=[-2*v1,(v1^2/v2)-v2;-2*v3,(v3^2/v4)-v4];
% D=(L1^2-L2^2)/L2;
% cos=D*(det(A)/det(C));
% sin=D*(det(B)/det(C));
% %%% After Including Zero Vector %%%
A=[(v3^2/v4)-v4,(i3-i01)-((v3/v4)*(i4-i02));(v1^2/v2)-v2,(i1-i01)-((v1/v2)*(i2-i02))];
B=[2*v3,(i3-i01)-((v3/v4)*(i4-i02));2*v1,(i1-i01)-((v1/v2)*(i2-i02))];
C=[-2*v1,(v1^2/v2)-v2;-2*v3,(v3^2/v4)-v4];
D=(L1^2-L2^2)/L2;
cos=D*(det(A)/det(C));
sin=D*(det(B)/det(C));

== matlab function sensorless/SVPWM3/MATLAB Function1 ==
  data: u input; y output
function y = fcn(u)
%#codegen
while u > 2*pi
    u = u-2*pi;
end
while u < 0
    u = u+2*pi;
end
y = u;

== matlab function sensorless/SVPWM3/MATLAB Function2 ==
  data: u input; y output
function y = fcn(u)
%#codegen
while u >= 2*pi
    u = u-2*pi;
end
while u < 0
    u = u+2*pi;
end
y = u;

== matlab function sensorless/dq-sixphasePMSM/Embedded MATLAB Function2 ==
  data: ia output; ialpha input; ibeta input; iz1 input; iz2 input; iz3 input; iz4 input; ib output; ic output; id output; ie output; if1 output
function [ia,ib,ic,id,ie,if1] = fcn(ialpha,ibeta,iz1,iz2,iz3,iz4)

%#eml
uxx=[ialpha,ibeta,iz1,iz2,iz3,iz4]';
T=1/sqrt(3)*[1 sqrt(3)/2 -1/2 -sqrt(3)/2 -1/2 0;
    0 1/2 sqrt(3)/2 1/2 -sqrt(3)/2 -1;
    1 -sqrt(3)/2 -1/2 sqrt(3)/2 -1/2 0;
    0 1/2 -sqrt(3)/2 1/2 sqrt(3)/2 -1;
    1 0 1 0 1 0;
    0 1 0 1 0 1];
I=inv(T)*uxx;
ia=I(1);
ib=I(2);
ic=I(3);
id=I(4);
ie=I(5);
if1=I(6);

== matlab function sensorless/SVPWM3/MATLAB Function4 ==
  data: x input; y output; clock input
function y = fcn(x,clock)
%#codegen

if clock<0.006
    y=0;
else
    y=x;
end
end

== matlab function sensorless/dq-sixphasePMSM/Embedded MATLAB Function3 ==
  data: ialpha input; id output; iq output; ibeta input; theta input
function [id,iq] = fcn(ialpha,ibeta,theta)

%#eml
uxx=[ialpha,ibeta]';
T=[cos(theta),-sin(theta);sin(theta),cos(theta)];
I=inv(T)*uxx;
id=I(1);
iq=I(2);

== matlab function sensorless/dq-sixphasePMSM/z-p/Subsystem/Manually Calculated Results  ==
  data: La0 input; Ld output; La1 input; Lg0 input; La2 input; Lg1 input; Lg2 input; RP input; Lq output; Lz1 output; Lz2 output; Lz1z2 output
function [Ld,Lq,Lz1,Lz2,Lz1z2] = fcn(La0,La1,Lg0,La2,Lg1,Lg2,RP)
%#codegen
Ld=3*La0+La1+sqrt(3)*La2+40*(1/2*Lg0+Lg1+Lg2);
Lq=3*La0+sqrt(3)*La2+La1-40*(1/2*Lg0+Lg1+Lg2);
Lz1=La1+cos(2*RP)*40*(1/2*Lg0-Lg1+Lg2)-sqrt(3)*La2;
Lz2=La1-cos(2*RP)*40*(1/2*Lg0-Lg1+Lg2)-sqrt(3)*La2;
Lz1z2=-sin(2*RP)*40*(1/2*Lg0-Lg1+Lg2);

== matlab function sensorless/dq-sixphasePMSM/z-p1/Subsystem/Manually Calculated Results  ==
  data: La0 input; Lalpha output; La1 input; Lg0 input; La2 input; Lg1 input; Lg2 input; RP input; Lbeta output; Lalphabeta output
function [Lalpha,Lbeta,Lalphabeta] = fcn(La0,La1,Lg0,La2,Lg1,Lg2,RP)
%#codegen
Lalpha=3*La0+La1+sqrt(3)*La2+40*(1/2*Lg0+Lg1+Lg2)*cos(2*RP);
Lbeta=3*La0+sqrt(3)*La2+La1-40*(1/2*Lg0+Lg1+Lg2)*cos(2*RP);
Lalphabeta=40*(1/2*Lg0+Lg1+Lg2)*sin(2*RP);

== matlab function sensorless/SVPWM3/Subsystem/frame Transformation for V1 abc-alpha_beta2 ==
  data: ia input; I_alpha_dV1 output; I_beta_dV1 output; ib input; ic input; id input; ie input; if1 input
function [I_alpha_dV1,I_beta_dV1]= fcn(ia,ib,ic,id,ie,if1)
%#codegen
d=[ia,ib,ic,id,ie,if1]';
C=1/sqrt(3)*[1 sqrt(3)/2 -1/2 -sqrt(3)/2 -1/2 0;
    0 1/2 sqrt(3)/2 1/2 -sqrt(3)/2 -1;
    1 -sqrt(3)/2 -1/2 sqrt(3)/2 -1/2 0;
    0 1/2 -sqrt(3)/2 1/2 sqrt(3)/2 -1;
    1 0 1 0 1 0;
    0 1 0 1 0 1];
h=C*d;
I_alpha_dV1=h(1,1);
I_beta_dV1=h(2,1);

== matlab function sensorless/SVPWM3/Subsystem/frame Transformation for V1 abc-alpha_beta3 ==
  data: ia input; I_alpha_dV1 output; I_beta_dV1 output; ib input; ic input; id input; ie input; if1 input
function [I_alpha_dV1,I_beta_dV1]= fcn(ia,ib,ic,id,ie,if1)
%#codegen
d=[ia,ib,ic,id,ie,if1]';
C=1/sqrt(3)*[1 sqrt(3)/2 -1/2 -sqrt(3)/2 -1/2 0;
    0 1/2 sqrt(3)/2 1/2 -sqrt(3)/2 -1;
    1 -sqrt(3)/2 -1/2 sqrt(3)/2 -1/2 0;
    0 1/2 -sqrt(3)/2 1/2 sqrt(3)/2 -1;
    1 0 1 0 1 0;
    0 1 0 1 0 1];
h=C*d;
I_alpha_dV1=h(1,1);
I_beta_dV1=h(2,1);

== matlab function sensorless/MATLAB Function3 ==
  data: u input; y output
function y = fcn(u)
%#codegen
if u<0.4
    y=30;
elseif u>1.3
    y=120;
else
    y=100*u-10;
end
end

== matlab function sensorless/SVPWM3/MATLAB Function6 ==
  data: s input; y output; s_delay1 input; s_delay2 input
function y = fcn(s,s_delay1,s_delay2)

if abs(s)<0.4
    y=s;
else
    if abs(s)>=0.4 && abs(s_delay1)<0.4
        y=s_delay1;
    else
        y=s_delay2;
    end
end
end

== matlab function sensorless/SVPWM3/Calculated Voltages /V_alpha1 & V_beta1 ==
  data: udc input; u_alpha1 output; N input; u_beta1 output
function [u_alpha1,u_beta1] = fcn(udc,N)
%#codegen
va01=0;%V49 
vb01=0;
va02=0;%V48
vb02=0;
va03=0;%V48
vb03=0;
va04=0;%V56
vb04=0;
va05=0;%V28
vb05=0;
va06=0;%V12
vb06=0;
va07=0;%V12
vb07=0;
va08=0;%V14
vb08=0;
va09=0;%V07
vb09=0;
va10=0;%V03
vb10=0;
va11=0;%V03
vb11=0;
va12=0;%V35
vb12=0;
u_alpha1=0;
u_beta1=0;
if N==1
va01=udc*1.115355072*cosd(345); 
vb01=udc*1.115355072*sind(345); 
u_alpha1=va01;
u_beta1=vb01;
end
if N==2
va02=udc*1.115355072*cosd(15);
vb02=udc*1.115355072*sind(15);
u_alpha1=va02;
u_beta1=vb02;
end
if N==3
va03=udc*1.115355072*cosd(15);
vb03=udc*1.115355072*sind(15);
u_alpha1=va03;
u_beta1=vb03;
end
if N==4
va04=udc*1.115355072*cosd(45);
vb04=udc*1.115355072*sind(45);
u_alpha1=va04;
u_beta1=vb04;
end
if N==5
va05=udc*1.115355072*cosd(105);
vb05=udc*1.115355072*sind(105);
u_alpha1=va05;
u_beta1=vb05;
end
if N==6
va06=udc*1.115355072*cosd(135);
vb06=udc*1.115355072*sind(135);
u_alpha1=va06;
u_beta1=vb06;
end
if N==7
va07=udc*1.115355072*cosd(135);
vb07=udc*1.115355072*sind(135);
u_alpha1=va07;
u_beta1=vb07;
end
if N==8
va08=udc*1.115355072*cosd(165);
vb08=udc*1.115355072*sind(165);
u_alpha1=va08;
u_beta1=vb08;
end
if N==9
va09=udc*1.115355072*cosd(225);
vb09=udc*1.115355072*sind(225);
u_alpha1=va09;
u_beta1=vb09;
end
if N==10
va10=udc*1.115355072*cosd(255);
vb10=udc*1.115355072*sind(255);
u_alpha1=va10;
u_beta1=vb10;
end
if N==11
va11=udc*1.115355072*cosd(255);
vb11=udc*1.115355072*sind(255);
u_alpha1=va11;
u_beta1=vb11;
end 
if N==12
va12=udc*1.115355072*cosd(285);
vb12=udc*1.115355072*sind(285);
u_alpha1=va12;
u_beta1=vb12;
end

== matlab function sensorless/MATLAB Function1 ==
  data: u input; y output
function y = fcn(u)
%#codegen
if u<0.6
    y=0;
elseif u>=0.6 && u<1.1
    y=50;
elseif u>=1.1 && u<1.6
    y=100;
elseif u>=1.6 && u<2.1
    y=50;
else
    y=0;
end
end

== matlab function sensorless/SVPWM3/MATLAB Function5 ==
  data: u input; y output
function y = fcn(u)
%#codegen
if u >180
    u = u-2*180;
end
if u <-180
    u = u+2*180;
end
y = u;

== matlab function sensorless/MATLAB Function4 ==
  data: u input; y output
function y = fcn(u)
%#codegen
if u<0.6
    y=0;
elseif u>=0.6 && u<1.2
    y=8;
elseif u>=1.2 && u<1.8
    y=16;
elseif u>=1.8 && u<2.4
    y=8;
else
    y=0;
end
end

== matlab function sensorless/SVPWM3/MATLAB Function7 ==
  data: s input; y output; s_delay1 input; s_delay2 input
function y = fcn(s,s_delay1,s_delay2)

if abs(s)<0.4
    y=s;
else
    if abs(s)>=0.4 && abs(s_delay1)<0.4
        y=s_delay1;
    else
        y=s_delay2;
    end
end
end

== matlab function sensorless/SVPWM3/MATLAB Function8 ==
  data: x input; y output
function y = fcn(x)
%#codegen
u=x+0.12;
while u > 2*pi
    u = u-2*pi;
end
while u < 0
    u = u+2*pi;
end
y = u;

== matlab function sensorless/SVPWM3/Embedded MATLAB Function2 ==
  data: ualpha1 output; ubeta1 output; ualpha2 output; ubeta2 output; N input; T1 output; Ualpha input; Ubeta input; Tpwm input; T2 output; T3 output; T4 output; T0 output; udc input; Uz1 input; Uz2 input
function [ualpha1,ubeta1,ualpha2,ubeta2,T1, T2, T3, T4, T0] = fcn(N, Ualpha, Ubeta, Tpwm, udc,Uz1,Uz2)
 m=sqrt(3)/2+1/2*i;                %等功率clarke反变换    
ab44=1/sqrt(3)*udc*[1,m^4,m^8,m,m^5,m^9]*[1;0;0;1;0;0];
xy44=1/sqrt(3)*udc*[1,m^8,m^4,m^5,m,m^9]*[1;0;0;1;0;0];

ab64=1/sqrt(3)*udc*[1,m^4,m^8,m,m^5,m^9]*[1;1;0;1;0;0];
xy64=1/sqrt(3)*udc*[1,m^8,m^4,m^5,m,m^9]*[1;1;0;1;0;0];
        
ab66=1/sqrt(3)*udc*[1,m^4,m^8,m,m^5,m^9]*[1;1;0;1;1;0];
xy66=1/sqrt(3)*udc*[1,m^8,m^4,m^5,m,m^9]*[1;1;0;1;1;0];

ab26=1/sqrt(3)*udc*[1,m^4,m^8,m,m^5,m^9]*[0;1;0;1;1;0];
xy26=1/sqrt(3)*udc*[1,m^8,m^4,m^5,m,m^9]*[0;1;0;1;1;0];

ab22=1/sqrt(3)*udc*[1,m^4,m^8,m,m^5,m^9]*[0;1;0;0;1;0];
xy22=1/sqrt(3)*udc*[1,m^8,m^4,m^5,m,m^9]*[0;1;0;0;1;0];

ab32=1/sqrt(3)*udc*[1,m^4,m^8,m,m^5,m^9]*[0;1;1;0;1;0];
xy32=1/sqrt(3)*udc*[1,m^8,m^4,m^5,m,m^9]*[0;1;1;0;1;0];

ab33=1/sqrt(3)*udc*[1,m^4,m^8,m,m^5,m^9]*[0;1;1;0;1;1];
xy33=1/sqrt(3)*udc*[1,m^8,m^4,m^5,m,m^9]*[0;1;1;0;1;1];

ab13=1/sqrt(3)*udc*[1,m^4,m^8,m,m^5,m^9]*[0;0;1;0;1;1];
xy13=1/sqrt(3)*udc*[1,m^8,m^4,m^5,m,m^9]*[0;0;1;0;1;1];

ab11=1/sqrt(3)*udc*[1,m^4,m^8,m,m^5,m^9]*[0;0;1;0;0;1];
xy11=1/sqrt(3)*udc*[1,m^8,m^4,m^5,m,m^9]*[0;0;1;0;0;1];

ab51=1/sqrt(3)*udc*[1,m^4,m^8,m,m^5,m^9]*[1;0;1;0;0;1];
xy51=1/sqrt(3)*udc*[1,m^8,m^4,m^5,m,m^9]*[1;0;1;0;0;1];

ab55=1/sqrt(3)*udc*[1,m^4,m^8,m,m^5,m^9]*[1;0;1;1;0;1];
xy55=1/sqrt(3)*udc*[1,m^8,m^4,m^5,m,m^9]*[1;0;1;1;0;1];

ab45=1/sqrt(3)*udc*[1,m^4,m^8,m,m^5,m^9]*[1;0;0;1;0;1];
xy45=1/sqrt(3)*udc*[1,m^8,m^4,m^5,m,m^9]*[1;0;0;1;0;1];

switch N
    case 1
        X=[real(ab55),real(ab45),real(ab44),real(ab64);
           imag(ab55),imag(ab45),imag(ab44),imag(ab64);
           real(xy55),real(xy45),real(xy44),real(xy64);
           imag(xy55),imag(xy45),imag(xy44),imag(xy64)];
       ualpha1=X(2,1);
       ubeta1=X(2,2);
       ualpha2=X(1,1);
       ubeta2=X(1,2);

    case 2
        X=[real(ab45),real(ab44),real(ab64),real(ab66);
           imag(ab45),imag(ab44),imag(ab64),imag(ab66);
           real(xy45),real(xy44),real(xy64),real(xy66);
           imag(xy45),imag(xy44),imag(xy64),imag(xy66)];
       ualpha1=X(2,1);
       ubeta1=X(2,2);
       ualpha2=X(1,1);
       ubeta2=X(1,2);
    case 3
        X=[real(ab44),real(ab64),real(ab66),real(ab26);
           imag(ab44),imag(ab64),imag(ab66),imag(ab26);
           real(xy44),real(xy64),real(xy66),real(xy26);
           imag(xy44),imag(xy64),imag(xy66),imag(xy26)];
       ualpha1=X(1,1);
       ubeta1=X(1,2);
       ualpha2=X(2,1);
       ubeta2=X(2,2);
    case 4
        X=[real(ab64),real(ab66),real(ab26),real(ab22);
           imag(ab64),imag(ab66),imag(ab26),imag(ab22);
           real(xy64),real(xy66),real(xy26),real(xy22);
           imag(xy64),imag(xy66),imag(xy26),imag(xy22)];
       ualpha1=X(1,1);
       ubeta1=X(1,2);
       ualpha2=X(2,1);
       ubeta2=X(2,2);
    case 5
        X=[real(ab66),real(ab26),real(ab22),real(ab32);
           imag(ab66),imag(ab26),imag(ab22),imag(ab32);
           real(xy66),real(xy26),real(xy22),real(xy32);
           imag(xy66),imag(xy26),imag(xy22),imag(xy32)];
       ualpha1=X(2,1);
       ubeta1=X(2,2);
       ualpha2=X(1,1);
       ubeta2=X(1,2);
    case 6
        X=[real(ab26),real(ab22),real(ab32),real(ab33);
           imag(ab26),imag(ab22),imag(ab32),imag(ab33);
           real(xy26),real(xy22),real(xy32),real(xy33);
           imag(xy26),imag(xy22),imag(xy32),imag(xy33)];
       ualpha1=X(2,1);
       ubeta1=X(2,2);
       ualpha2=X(1,1);
       ubeta2=X(1,2);
    case 7
        X=[real(ab22),real(ab32),real(ab33),real(ab13);
           imag(ab22),imag(ab32),imag(ab33),imag(ab13);
           real(xy22),real(xy32),real(xy33),real(xy13);
           imag(xy22),imag(xy32),imag(xy33),imag(xy13)];
       ualpha1=X(1,1);
       ubeta1=X(1,2);
       ualpha2=X(2,1);
       ubeta2=X(2,2);
    case 8
        X=[real(ab32),real(ab33),real(ab13),real(ab11);
           imag(ab32),imag(ab33),imag(ab13),imag(ab11);
           real(xy32),real(xy33),real(xy13),real(xy11);
           imag(xy32),imag(xy33),imag(xy13),imag(xy11)];
       ualpha1=X(1,1);
       ubeta1=X(1,2);
       ualpha2=X(2,1);
       ubeta2=X(2,2);
    case 9
        X=[real(ab33),real(ab13),real(ab11),real(ab51);
           imag(ab33),imag(ab13),imag(ab11),imag(ab51);
           real(xy33),real(xy13),real(xy11),real(xy51);
           imag(xy33),imag(xy13),imag(xy11),imag(xy51)];
       ualpha1=X(2,1);
       ubeta1=X(2,2);
       ualpha2=X(1,1);
       ubeta2=X(1,2);
    case 10
        X=[real(ab13),real(ab11),real(ab51),real(ab55);
           imag(ab13),imag(ab11),imag(ab51),imag(ab55);
           real(xy13),real(xy11),real(xy51),real(xy55);
           imag(xy13),imag(xy11),imag(xy51),imag(xy55)];
       ualpha1=X(2,1);
       ubeta1=X(2,2);
       ualpha2=X(1,1);
       ubeta2=X(1,2);
    case 11
        X=[real(ab11),real(ab51),real(ab55),real(ab45);
           imag(ab11),imag(ab51),imag(ab55),imag(ab45);
           real(xy11),real(xy51),real(xy55),real(xy45);
           imag(xy11),imag(xy51),imag(xy55),imag(xy45)];
       ualpha1=X(1,1);
       ubeta1=X(1,2);
       ualpha2=X(2,1);
       ubeta2=X(2,2);
    case 12
        X=[real(ab51),real(ab55),real(ab45),real(ab44);
           imag(ab51),imag(ab55),imag(ab45),imag(ab44);
           real(xy51),real(xy55),real(xy45),real(xy44);
           imag(xy51),imag(xy55),imag(xy45),imag(xy44)];
       ualpha1=X(1,1);
       ubeta1=X(1,2);
       ualpha2=X(2,1);
       ubeta2=X(2,2);
    otherwise
        X=[0,0,0,0;
           0,0,0,0;
           0,0,0,0;
           0,0,0,0];
       ualpha1=X(1,1);
       ubeta1=X(1,2);
       ualpha2=X(2,1);
       ubeta2=X(2,2);
end
Y=[Ualpha;Ubeta;Uz1;Uz2]*Tpwm;
T=inv(X)*Y;
show=X*T;
u1=1/Tpwm*show(1);
u2=1/Tpwm*show(2);
u3=1/Tpwm*show(3);
u4=1/Tpwm*show(4);


T1=T(1);
if T1<1e-6
    T1=1e-6;
end 
T2=T(2);
if T2<1e-6
    T2=1e-6;
end 
T3=T(3);
if T3<1e-6
    T3=1e-6;
end 
T4=T(4);
if T4<1e-6
    T4=1e-6;
end
% T1=T(1);
% T2=T(2);
% T3=T(3);
% T4=T(4);
Tsum=T1+T2+T3+T4;
if Tsum>Tpwm
    T1=T1*Tpwm/Tsum;
    T2=T2*Tpwm/Tsum;
    T3=T3*Tpwm/Tsum;
    T4=T4*Tpwm/Tsum;
end
T0=Tpwm-T1-T2-T3-T4;
end

== matlab function sensorless/SVPWM3/Embedded MATLAB Function6 ==
  data: N output; ualfa input; ubeta input; TH output
function [N,TH] = fcn(ualfa,ubeta)

%#xsxx
[TH,R] = cart2pol(ualfa,ubeta);
if TH<0
    TH=TH+2*pi;
end
N=floor((TH+pi/12)/(pi/6))+1;
if N==13
    N=1;
end;
%N=floor((TH)/(pi/3))+1;

== matlab function sensorless/SVPWM3/MATLAB Function9 ==
  data: s input; y output; s_delay1 input
function y = fcn(s,s_delay1)

if abs(s-s_delay1)<0.02
    y=s;
else
    y=s_delay1;
end
end

== matlab function sensorless/SVPWM3/rest of others ==
  data: N input; T1 input; T2 input; T3 input; T4 input; T0 input; Tcma1 output; Tcma2 output; Tcmb1 output; Tcmb2 output; Tcmc1 output; Tcmc2 output; Tcmd1 output; Tcmd2 output; Tcme1 output; Tcme2 output; Tcmf1 output; Tcmf2 output
function [Tcma1,Tcma2,Tcmb1,Tcmb2,Tcmc1,Tcmc2,Tcmd1,Tcmd2,Tcme1,Tcme2,Tcmf1,Tcmf2] = fcn(N,T1,T2,T3,T4,T0)

%#xsxx
Ta=T0/4;
Tb=Ta+T2;
Tc=Tb+T1;
Td=Tc+T0/2;
Te=Td+T4;
Tf=Te+T3;

Ta1=T0/4;
Tb1=Ta1+T1;
Tc1=Tb1+T2;
Td1=Tc1+T0/2;
Te1=Td1+T3;
Tf1=Te1+T4;

Tcma1=0;
Tcma2=0;
Tcmb1=0;
Tcmb2=0;
Tcmc1=0;
Tcmc2=0;
Tcmd1=0;
Tcmd2=0;
Tcme1=0;
Tcme2=0;
Tcmf1=0;
Tcmf2=0;
if N==1
    Tcma1=Ta;%TIme of "00" voltage vector 
    Tcma2=Tf;%TIme of "48" voltage vector 
    Tcmb1=Ta;
    Tcmb2=Tf;
    Tcmc1=Tc;%TIme of "51" voltage vector 
    Tcmc2=Te;%TIme of "56" voltage vector 
    Tcmd1=Tc;
    Tcmd2=Td;
    Tcme1=Tb;%TIme of "49" voltage vector 
    Tcme2=Td;%TIme of "63" voltage vector 
    Tcmf1=Ta;
    Tcmf2=Td;
elseif N==2
    Tcma1=Ta;
    Tcma2=Tf;
    Tcmb1=Ta;
    Tcmb2=Tf;
    Tcmc1=Tc;
    Tcmc2=Tf;
    Tcmd1=Tc;
    Tcmd2=Te;
    Tcme1=Tc;
    Tcme2=Td;
    Tcmf1=Tb;
    Tcmf2=Td;
elseif N==3
    Tcma1=Ta1;
    Tcma2=Te1;
    Tcmb1=Ta1;
    Tcmb2=Tf1;
    Tcmc1=Tb1;
    Tcmc2=Tf1;
    Tcmd1=Tc1;
    Tcmd2=Tf1;
    Tcme1=Tc1;
    Tcme2=Td1;
    Tcmf1=Tc1;
    Tcmf2=Td1;
elseif N==4
    Tcma1=Ta1;
    Tcma2=Td1;
    Tcmb1=Ta1;
    Tcmb2=Te1;
    Tcmc1=Ta1;
    Tcmc2=Tf1;
    Tcmd1=Tb1;
    Tcmd2=Tf1;
    Tcme1=Tc1;
    Tcme2=Td1;
    Tcmf1=Tc1;
    Tcmf2=Td1;
elseif N==5
    Tcma1=Tb;
    Tcma2=Td;
    Tcmb1=Ta;
    Tcmb2=Td;
    Tcmc1=Ta;
    Tcmc2=Tf;
    Tcmd1=Ta;
    Tcmd2=Tf;
    Tcme1=Tc;
    Tcme2=Te;
    Tcmf1=Tc;
    Tcmf2=Td;
elseif N==6
    Tcma1=Tc;
    Tcma2=Td;
    Tcmb1=Tb;
    Tcmb2=Td;
    Tcmc1=Ta;
    Tcmc2=Tf;
    Tcmd1=Ta;
    Tcmd2=Tf;
    Tcme1=Tc;
    Tcme2=Tf;
    Tcmf1=Tc;
    Tcmf2=Te;
elseif N==7
    Tcma1=Tc1;
    Tcma2=Td1;
    Tcmb1=Tc1;
    Tcmb2=Td1;
    Tcmc1=Ta1;
    Tcmc2=Te1;
    Tcmd1=Ta1;
    Tcmd2=Tf1;
    Tcme1=Tb1;
    Tcme2=Tf1;
    Tcmf1=Tc1;
    Tcmf2=Tf1;
elseif N==8
    Tcma1=Tc1;
    Tcma2=Td1;
    Tcmb1=Tc1;
    Tcmb2=Td1;
    Tcmc1=Ta1;
    Tcmc2=Td1;
    Tcmd1=Ta1;
    Tcmd2=Te1;
    Tcme1=Ta1;
    Tcme2=Tf1;
    Tcmf1=Tb1;
    Tcmf2=Tf1;
elseif N==9
    Tcma1=Tc;
    Tcma2=Te;
    Tcmb1=Tc;
    Tcmb2=Td;
    Tcmc1=Tb;
    Tcmc2=Td;
    Tcmd1=Ta;
    Tcmd2=Td;
    Tcme1=Ta;
    Tcme2=Tf;
    Tcmf1=Ta;
    Tcmf2=Tf;
elseif N==10
    Tcma1=Tc;
    Tcma2=Tf;
    Tcmb1=Tc;
    Tcmb2=Te;
    Tcmc1=Tc;
    Tcmc2=Td;
    Tcmd1=Tb;
    Tcmd2=Td;
    Tcme1=Ta;
    Tcme2=Tf;
    Tcmf1=Ta;
    Tcmf2=Tf;
elseif N==11
    Tcma1=Tb1;
    Tcma2=Tf1;
    Tcmb1=Tc1;
    Tcmb2=Tf1;
    Tcmc1=Tc1;
    Tcmc2=Td1;
    Tcmd1=Tc1;
    Tcmd2=Td1;
    Tcme1=Ta1;
    Tcme2=Te1;
    Tcmf1=Ta1;
    Tcmf2=Tf1;
elseif N==12
    Tcma1=Ta1;
    Tcma2=Tf1;
    Tcmb1=Tb1;
    Tcmb2=Tf1;
    Tcmc1=Tc1;
    Tcmc2=Td1;
    Tcmd1=Tc1;
    Tcmd2=Td1;
    Tcme1=Ta1;
    Tcme2=Td1;
    Tcmf1=Ta1;
    Tcmf2=Te1;
end

== matlab function sensorless/SVPWM3/MATLAB Function10 ==
  data: s input; y output; s_delay1 input
function y = fcn(s,s_delay1)

if abs(s-s_delay1)<0.02
    y=s;
else
    y=s_delay1;
end
end

== matlab function sensorless/SVPWM3/MATLAB Function11 ==
  data: u input; y output
function y = fcn(u)
%#codegen
if u >360
    u = u-2*180;
end
if u <0
    u = u+2*180;
end
y = u;
